simulink model "c00014M_harness"  (R2018a)
settings: Solver=FixedStepAuto  StartTime=0.0  StopTime=300  FixedStep=0.1  RelTol=1e-3
undefined symbols (not defined in the file): A1, hmax, PriorityTank, R1, R2, sigbuilder_block
(part 13 of 24)

== system c00014M_harness/M144/Tank1/Control ==
  note: 1: Maintenance
      | 2: Reference
      | 3: Manual
  ControlType : Inport
  Fill : Inport  Port=2
  Empty : Inport  Port=3
  EmergencyButton : Inport  Port=4
  LiquidLevel : Inport  Port=5
  Constant : Constant  Value=0
  ManualControlLiquidInOut : Subsystem
  Switch : Switch  Criteria=u2 > Threshold
  Switch1 : Switch  Criteria=u2 > Threshold
  LiquidIn : Outport
  LiquidOut : Outport  Port=2
  wires:
  LiquidLevel/1 -> ManualControlLiquidInOut/3(LiquidLevel)
  Empty/1 -> ManualControlLiquidInOut/2(Empty)
  Fill/1 -> ManualControlLiquidInOut/1(Fill)
  Switch/1 -> LiquidIn/1
  Switch1/1 -> LiquidOut/1
  Constant/1 -> Switch1/1, Switch/1
  EmergencyButton/1 -> Switch/2, Switch1/2
  ManualControlLiquidInOut/1(LiquidIn) -> Switch/3
  ManualControlLiquidInOut/2(LiquidOut) -> Switch1/3

== system c00014M_harness/M144/Tank1/MasterTankControl ==
  note: Priority tank must always have more liquid than others
  LiquidTank1 : Inport
  LiquidTank3 : Inport  Port=2
  Constant : Constant  Value=PriorityTank
  Constant1 : Constant  Value=false
  Logical Operator : Logic  Operator=NOT  AllPortsSameDT=off  OutDataTypeStr=boolean
  Multiport Switch : MultiPortSwitch
  Relational Operator1 : RelationalOperator  OutDataTypeStr=boolean  RndMeth=Simplest
  AllowTheTankFilling : Outport
  wires:
  LiquidTank3/1 -> Relational Operator1/2
  LiquidTank1/1 -> Relational Operator1/1
  Constant/1 -> Multiport Switch/1
  Relational Operator1/1 -> Multiport Switch/4
  Constant1/1 -> Multiport Switch/2, Multiport Switch/3
  Multiport Switch/1 -> Logical Operator/1
  Logical Operator/1 -> AllowTheTankFilling/1

== system c00014M_harness/M144/Tank1/TankModel ==
  LiquidIn : Inport
  LiquidOut : Inport  Port=2
  Add1 : Sum  Inputs=+-
  Constant1 : Constant  Value=0
  Constant2 : Constant  Value=0
  Constant3 : Constant
  Gain : Gain  Gain=1/R1
  Gain1 : Gain  Gain=1/A1
  Gain2 : Gain  Gain=1/R2
  Integrator : Integrator
  Saturation : Saturate  UpperLimit=hmax  LowerLimit=0
  Switch : Switch  Criteria=u2 ~= 0
  Switch1 : Switch  Criteria=u2 ~= 0
  LiquidLevel : Outport
  wires:
  Saturation/1 -> LiquidLevel/1, Gain2/1
  LiquidOut/1 -> Switch/2
  Add1/1 -> Gain1/1
  Gain2/1 -> Switch/1
  LiquidIn/1 -> Switch1/2
  Switch/1 -> Add1/2
  Switch1/1 -> Gain/1
  Constant2/1 -> Switch/3
  Constant3/1 -> Switch1/1
  Integrator/1 -> Saturation/1
  Gain1/1 -> Integrator/1
  Gain/1 -> Add1/1
  Constant1/1 -> Switch1/3

== system c00014M_harness/M144/Tank3/Control ==
  note: 1: Maintenance
      | 2: Reference
      | 3: Manual
  ControlType : Inport
  StartMaintenance : Inport  Port=2
  EmergencyButton : Inport  Port=3
  LiquidLevel : Inport  Port=4
  Constant : Constant  Value=0
  Maintenance : Subsystem
  Switch : Switch  Criteria=u2 > Threshold
  Switch1 : Switch  Criteria=u2 > Threshold
  LiquidIn : Outport
  LiquidOut : Outport  Port=2
  wires:
  ControlType/1 -> Maintenance/1(Type)
  LiquidLevel/1 -> Maintenance/3(LiquidLevel)
  StartMaintenance/1 -> Maintenance/2(StartMaintenance)
  Switch/1 -> LiquidIn/1
  Switch1/1 -> LiquidOut/1
  Constant/1 -> Switch1/1, Switch/1
  EmergencyButton/1 -> Switch/2, Switch1/2
  Maintenance/1(LiquidIn) -> Switch/3
  Maintenance/2(LiquidOut) -> Switch1/3

== system c00014M_harness/M144/Tank3/MasterTankControl ==
  note: Priority tank must always have more liquid than others
  LiquidTank1 : Inport
  LiquidTank3 : Inport  Port=2
  Constant : Constant  Value=PriorityTank
  Constant1 : Constant  Value=false
  Logical Operator : Logic  Operator=NOT  AllPortsSameDT=off  OutDataTypeStr=boolean
  Multiport Switch : MultiPortSwitch
  Relational Operator : RelationalOperator  OutDataTypeStr=boolean  RndMeth=Simplest
  AllowTheTankFilling : Outport
  wires:
  Constant/1 -> Multiport Switch/1
  Relational Operator/1 -> Multiport Switch/2
  Constant1/1 -> Multiport Switch/4, Multiport Switch/3
  Multiport Switch/1 -> Logical Operator/1
  Logical Operator/1 -> AllowTheTankFilling/1
  LiquidTank1/1 -> Relational Operator/2
  LiquidTank3/1 -> Relational Operator/1

== system c00014M_harness/M144/Tank3/TankModel ==
  LiquidIn : Inport
  LiquidOut : Inport  Port=2
  Add1 : Sum  Inputs=+-
  Constant1 : Constant  Value=0
  Constant2 : Constant  Value=0
  Constant3 : Constant
  Gain : Gain  Gain=1/R1
  Gain1 : Gain  Gain=1/A1
  Gain2 : Gain  Gain=1/R2
  Integrator : Integrator
  Saturation : Saturate  UpperLimit=hmax  LowerLimit=0
  Switch : Switch  Criteria=u2 ~= 0
  Switch1 : Switch  Criteria=u2 ~= 0
  LiquidLevel : Outport
  wires:
  Saturation/1 -> LiquidLevel/1, Gain2/1
  LiquidOut/1 -> Switch/2
  Add1/1 -> Gain1/1
  Gain2/1 -> Switch/1
  LiquidIn/1 -> Switch1/2
  Switch/1 -> Add1/2
  Switch1/1 -> Gain/1
  Constant2/1 -> Switch/3
  Constant3/1 -> Switch1/1
  Integrator/1 -> Saturation/1
  Gain1/1 -> Integrator/1
  Gain/1 -> Add1/1
  Constant1/1 -> Switch1/3

== system c00014M_harness/M145/Tank1/Control ==
  note: 1: Maintenance
      | 2: Reference
      | 3: Manual
  ControlType : Inport
  Fill : Inport  Port=2
  Empty : Inport  Port=3
  EmergencyButton : Inport  Port=4
  LiquidLevel : Inport  Port=5
  Constant : Constant  Value=0
  ManualControlLiquidInOut : Subsystem
  Switch : Switch  Criteria=u2 > Threshold
  Switch1 : Switch  Criteria=u2 > Threshold
  LiquidIn : Outport
  LiquidOut : Outport  Port=2
  wires:
  LiquidLevel/1 -> ManualControlLiquidInOut/3(LiquidLevel)
  Empty/1 -> ManualControlLiquidInOut/2(Empty)
  Fill/1 -> ManualControlLiquidInOut/1(Fill)
  Switch/1 -> LiquidIn/1
  Switch1/1 -> LiquidOut/1
  Constant/1 -> Switch1/1, Switch/1
  EmergencyButton/1 -> Switch/2, Switch1/2
  ManualControlLiquidInOut/1(LiquidIn) -> Switch/3
  ManualControlLiquidInOut/2(LiquidOut) -> Switch1/3

== system c00014M_harness/M145/Tank1/MasterTankControl ==
  note: Priority tank must always have more liquid than others
  LiquidTank1 : Inport
  LiquidTank3 : Inport  Port=2
  Constant : Constant  Value=PriorityTank
  Constant1 : Constant  Value=false
  Logical Operator : Logic  Operator=NOT  AllPortsSameDT=off  OutDataTypeStr=boolean
  Multiport Switch : MultiPortSwitch
  Relational Operator1 : RelationalOperator  OutDataTypeStr=boolean  RndMeth=Simplest
  AllowTheTankFilling : Outport
  wires:
  LiquidTank3/1 -> Relational Operator1/2
  LiquidTank1/1 -> Relational Operator1/1
  Constant/1 -> Multiport Switch/1
  Relational Operator1/1 -> Multiport Switch/4
  Constant1/1 -> Multiport Switch/2, Multiport Switch/3
  Multiport Switch/1 -> Logical Operator/1
  Logical Operator/1 -> AllowTheTankFilling/1

== system c00014M_harness/M145/Tank1/TankModel ==
  LiquidIn : Inport
  LiquidOut : Inport  Port=2
  Add1 : Sum  Inputs=+-
  Constant1 : Constant  Value=0
  Constant2 : Constant  Value=0
  Constant3 : Constant
  Gain : Gain  Gain=1/R1
  Gain1 : Gain  Gain=1/A1
  Gain2 : Gain  Gain=1/R2
  Integrator : Integrator
  Saturation : Saturate  UpperLimit=hmax  LowerLimit=0
  Switch : Switch  Criteria=u2 ~= 0
  Switch1 : Switch  Criteria=u2 ~= 0
  LiquidLevel : Outport
  wires:
  Saturation/1 -> LiquidLevel/1, Gain2/1
  LiquidOut/1 -> Switch/2
  Add1/1 -> Gain1/1
  Gain2/1 -> Switch/1
  LiquidIn/1 -> Switch1/2
  Switch/1 -> Add1/2
  Switch1/1 -> Gain/1
  Constant2/1 -> Switch/3
  Constant3/1 -> Switch1/1
  Integrator/1 -> Saturation/1
  Gain1/1 -> Integrator/1
  Gain/1 -> Add1/1
  Constant1/1 -> Switch1/3

== system c00014M_harness/M145/Tank3/Control ==
  note: 1: Maintenance
      | 2: Reference
      | 3: Manual
  ControlType : Inport
  StartMaintenance : Inport  Port=2
  EmergencyButton : Inport  Port=3
  LiquidLevel : Inport  Port=4
  Constant : Constant  Value=0
  Maintenance : Subsystem
  Switch : Switch  Criteria=u2 > Threshold
  Switch1 : Switch  Criteria=u2 > Threshold
  LiquidIn : Outport
  LiquidOut : Outport  Port=2
  wires:
  ControlType/1 -> Maintenance/1(Type)
  LiquidLevel/1 -> Maintenance/3(LiquidLevel)
  StartMaintenance/1 -> Maintenance/2(StartMaintenance)
  Switch/1 -> LiquidIn/1
  Switch1/1 -> LiquidOut/1
  Constant/1 -> Switch1/1, Switch/1
  EmergencyButton/1 -> Switch/2, Switch1/2
  Maintenance/1(LiquidIn) -> Switch/3
  Maintenance/2(LiquidOut) -> Switch1/3

== system c00014M_harness/M145/Tank3/MasterTankControl ==
  note: Priority tank must always have more liquid than others
  LiquidTank1 : Inport
  LiquidTank3 : Inport  Port=2
  Constant : Constant  Value=PriorityTank
  Constant1 : Constant  Value=false
  Logical Operator : Logic  Operator=NOT  AllPortsSameDT=off  OutDataTypeStr=boolean
  Multiport Switch : MultiPortSwitch
  Relational Operator : RelationalOperator  OutDataTypeStr=boolean  RndMeth=Simplest
  AllowTheTankFilling : Outport
  wires:
  Constant/1 -> Multiport Switch/1
  Relational Operator/1 -> Multiport Switch/2
  Constant1/1 -> Multiport Switch/4, Multiport Switch/3
  Multiport Switch/1 -> Logical Operator/1
  Logical Operator/1 -> AllowTheTankFilling/1
  LiquidTank1/1 -> Relational Operator/2
  LiquidTank3/1 -> Relational Operator/1

== system c00014M_harness/M145/Tank3/TankModel ==
  LiquidIn : Inport
  LiquidOut : Inport  Port=2
  Add1 : Sum  Inputs=+-
  Constant1 : Constant  Value=0
  Constant2 : Constant  Value=0
  Constant3 : Constant
  Gain : Gain  Gain=1/R1
  Gain1 : Gain  Gain=1/A1
  Gain2 : Gain  Gain=1/R2
  Integrator : Integrator
  Saturation : Saturate  UpperLimit=hmax  LowerLimit=0
  Switch : Switch  Criteria=u2 ~= 0
  Switch1 : Switch  Criteria=u2 ~= 0
  LiquidLevel : Outport
  wires:
  Saturation/1 -> LiquidLevel/1, Gain2/1
  LiquidOut/1 -> Switch/2
  Add1/1 -> Gain1/1
  Gain2/1 -> Switch/1
  LiquidIn/1 -> Switch1/2
  Switch/1 -> Add1/2
  Switch1/1 -> Gain/1
  Constant2/1 -> Switch/3
  Constant3/1 -> Switch1/1
  Integrator/1 -> Saturation/1
  Gain1/1 -> Integrator/1
  Gain/1 -> Add1/1
  Constant1/1 -> Switch1/3

== system c00014M_harness/M146/Tank1/Control ==
  note: 1: Maintenance
      | 2: Reference
      | 3: Manual
  ControlType : Inport
  Fill : Inport  Port=2
  Empty : Inport  Port=3
  EmergencyButton : Inport  Port=4
  LiquidLevel : Inport  Port=5
  Constant : Constant  Value=0
  ManualControlLiquidInOut : Subsystem
  Switch : Switch  Criteria=u2 > Threshold
  Switch1 : Switch  Criteria=u2 > Threshold
  LiquidIn : Outport
  LiquidOut : Outport  Port=2
  wires:
  LiquidLevel/1 -> ManualControlLiquidInOut/3(LiquidLevel)
  Empty/1 -> ManualControlLiquidInOut/2(Empty)
  Fill/1 -> ManualControlLiquidInOut/1(Fill)
  Switch/1 -> LiquidIn/1
  Switch1/1 -> LiquidOut/1
  Constant/1 -> Switch1/1, Switch/1
  EmergencyButton/1 -> Switch/2, Switch1/2
  ManualControlLiquidInOut/1(LiquidIn) -> Switch/3
  ManualControlLiquidInOut/2(LiquidOut) -> Switch1/3

== system c00014M_harness/M146/Tank1/MasterTankControl ==
  note: Priority tank must always have more liquid than others
  LiquidTank1 : Inport
  LiquidTank3 : Inport  Port=2
  Constant : Constant  Value=PriorityTank
  Constant1 : Constant  Value=false
  Logical Operator : Logic  Operator=NOT  AllPortsSameDT=off  OutDataTypeStr=boolean
  Multiport Switch : MultiPortSwitch
  Relational Operator1 : RelationalOperator  OutDataTypeStr=boolean  RndMeth=Simplest
  AllowTheTankFilling : Outport
  wires:
  LiquidTank3/1 -> Relational Operator1/2
  LiquidTank1/1 -> Relational Operator1/1
  Constant/1 -> Multiport Switch/1
  Relational Operator1/1 -> Multiport Switch/4
  Constant1/1 -> Multiport Switch/2, Multiport Switch/3
  Multiport Switch/1 -> Logical Operator/1
  Logical Operator/1 -> AllowTheTankFilling/1

== system c00014M_harness/M146/Tank1/TankModel ==
  LiquidIn : Inport
  LiquidOut : Inport  Port=2
  Add1 : Sum  Inputs=+-
  Constant1 : Constant  Value=0
  Constant2 : Constant  Value=0
  Constant3 : Constant
  Gain : Gain  Gain=1/R1
  Gain1 : Gain  Gain=1/A1
  Gain2 : Gain  Gain=1/R2
  Integrator : Integrator
  Saturation : Saturate  UpperLimit=hmax  LowerLimit=0
  Switch : Switch  Criteria=u2 ~= 0
  Switch1 : Switch  Criteria=u2 ~= 0
  LiquidLevel : Outport
  wires:
  Saturation/1 -> LiquidLevel/1, Gain2/1
  LiquidOut/1 -> Switch/2
  Add1/1 -> Gain1/1
  Gain2/1 -> Switch/1
  LiquidIn/1 -> Switch1/2
  Switch/1 -> Add1/2
  Switch1/1 -> Gain/1
  Constant2/1 -> Switch/3
  Constant3/1 -> Switch1/1
  Integrator/1 -> Saturation/1
  Gain1/1 -> Integrator/1
  Gain/1 -> Add1/1
  Constant1/1 -> Switch1/3

== system c00014M_harness/M146/Tank3/Control ==
  note: 1: Maintenance
      | 2: Reference
      | 3: Manual
  ControlType : Inport
  StartMaintenance : Inport  Port=2
  EmergencyButton : Inport  Port=3
  LiquidLevel : Inport  Port=4
  Constant : Constant  Value=0
  Maintenance : Subsystem
  Switch : Switch  Criteria=u2 > Threshold
  Switch1 : Switch  Criteria=u2 > Threshold
  LiquidIn : Outport
  LiquidOut : Outport  Port=2
  wires:
  ControlType/1 -> Maintenance/1(Type)
  LiquidLevel/1 -> Maintenance/3(LiquidLevel)
  StartMaintenance/1 -> Maintenance/2(StartMaintenance)
  Switch/1 -> LiquidIn/1
  Switch1/1 -> LiquidOut/1
  Constant/1 -> Switch1/1, Switch/1
  EmergencyButton/1 -> Switch/2, Switch1/2
  Maintenance/1(LiquidIn) -> Switch/3
  Maintenance/2(LiquidOut) -> Switch1/3

== system c00014M_harness/M146/Tank3/MasterTankControl ==
  note: Priority tank must always have more liquid than others
  LiquidTank1 : Inport
  LiquidTank3 : Inport  Port=2
  Constant : Constant  Value=PriorityTank
  Constant1 : Constant  Value=false
  Logical Operator : Logic  Operator=NOT  AllPortsSameDT=off  OutDataTypeStr=boolean
  Multiport Switch : MultiPortSwitch
  Relational Operator : RelationalOperator  OutDataTypeStr=boolean  RndMeth=Simplest
  AllowTheTankFilling : Outport
  wires:
  Constant/1 -> Multiport Switch/1
  Relational Operator/1 -> Multiport Switch/2
  Constant1/1 -> Multiport Switch/4, Multiport Switch/3
  Multiport Switch/1 -> Logical Operator/1
  Logical Operator/1 -> AllowTheTankFilling/1
  LiquidTank1/1 -> Relational Operator/2
  LiquidTank3/1 -> Relational Operator/1

== system c00014M_harness/M146/Tank3/TankModel ==
  LiquidIn : Inport
  LiquidOut : Inport  Port=2
  Add1 : Sum  Inputs=+-
  Constant1 : Constant  Value=0
  Constant2 : Constant  Value=0
  Constant3 : Constant
  Gain : Gain  Gain=1/R1
  Gain1 : Gain  Gain=1/A1
  Gain2 : Gain  Gain=1/R2
  Integrator : Integrator
  Saturation : Saturate  UpperLimit=hmax  LowerLimit=0
  Switch : Switch  Criteria=u2 ~= 0
  Switch1 : Switch  Criteria=u2 ~= 0
  LiquidLevel : Outport
  wires:
  Saturation/1 -> LiquidLevel/1, Gain2/1
  LiquidOut/1 -> Switch/2
  Add1/1 -> Gain1/1
  Gain2/1 -> Switch/1
  LiquidIn/1 -> Switch1/2
  Switch/1 -> Add1/2
  Switch1/1 -> Gain/1
  Constant2/1 -> Switch/3
  Constant3/1 -> Switch1/1
  Integrator/1 -> Saturation/1
  Gain1/1 -> Integrator/1
  Gain/1 -> Add1/1
  Constant1/1 -> Switch1/3

== system c00014M_harness/M147/Tank1/Control ==
  note: 1: Maintenance
      | 2: Reference
      | 3: Manual
  ControlType : Inport
  Fill : Inport  Port=2
  Empty : Inport  Port=3
  EmergencyButton : Inport  Port=4
  LiquidLevel : Inport  Port=5
  Constant : Constant  Value=0
  ManualControlLiquidInOut : Subsystem
  Switch : Switch  Criteria=u2 > Threshold
  Switch1 : Switch  Criteria=u2 > Threshold
  LiquidIn : Outport
  LiquidOut : Outport  Port=2
  wires:
  LiquidLevel/1 -> ManualControlLiquidInOut/3(LiquidLevel)
  Empty/1 -> ManualControlLiquidInOut/2(Empty)
  Fill/1 -> ManualControlLiquidInOut/1(Fill)
  Switch/1 -> LiquidIn/1
  Switch1/1 -> LiquidOut/1
  Constant/1 -> Switch1/1, Switch/1
  EmergencyButton/1 -> Switch/2, Switch1/2
  ManualControlLiquidInOut/1(LiquidIn) -> Switch/3
  ManualControlLiquidInOut/2(LiquidOut) -> Switch1/3

== system c00014M_harness/M147/Tank1/MasterTankControl ==
  note: Priority tank must always have more liquid than others
  LiquidTank1 : Inport
  LiquidTank3 : Inport  Port=2
  Constant : Constant  Value=PriorityTank
  Constant1 : Constant  Value=false
  Logical Operator : Logic  Operator=NOT  AllPortsSameDT=off  OutDataTypeStr=boolean
  Multiport Switch : MultiPortSwitch
  Relational Operator1 : RelationalOperator  OutDataTypeStr=boolean  RndMeth=Simplest
  AllowTheTankFilling : Outport
  wires:
  LiquidTank3/1 -> Relational Operator1/2
  LiquidTank1/1 -> Relational Operator1/1
  Constant/1 -> Multiport Switch/1
  Relational Operator1/1 -> Multiport Switch/4
  Constant1/1 -> Multiport Switch/2, Multiport Switch/3
  Multiport Switch/1 -> Logical Operator/1
  Logical Operator/1 -> AllowTheTankFilling/1

== system c00014M_harness/M147/Tank1/TankModel ==
  LiquidIn : Inport
  LiquidOut : Inport  Port=2
  Add1 : Sum  Inputs=+-
  Constant1 : Constant  Value=0
  Constant2 : Constant  Value=0
  Constant3 : Constant
  Gain : Gain  Gain=1/R1
  Gain1 : Gain  Gain=1/A1
  Gain2 : Gain  Gain=1/R2
  Integrator : Integrator
  Saturation : Saturate  UpperLimit=hmax  LowerLimit=0
  Switch : Switch  Criteria=u2 ~= 0
  Switch1 : Switch  Criteria=u2 ~= 0
  LiquidLevel : Outport
  wires:
  Saturation/1 -> LiquidLevel/1, Gain2/1
  LiquidOut/1 -> Switch/2
  Add1/1 -> Gain1/1
  Gain2/1 -> Switch/1
  LiquidIn/1 -> Switch1/2
  Switch/1 -> Add1/2
  Switch1/1 -> Gain/1
  Constant2/1 -> Switch/3
  Constant3/1 -> Switch1/1
  Integrator/1 -> Saturation/1
  Gain1/1 -> Integrator/1
  Gain/1 -> Add1/1
  Constant1/1 -> Switch1/3

== system c00014M_harness/M147/Tank3/Control ==
  note: 1: Maintenance
      | 2: Reference
      | 3: Manual
  ControlType : Inport
  StartMaintenance : Inport  Port=2
  EmergencyButton : Inport  Port=3
  LiquidLevel : Inport  Port=4
  Constant : Constant  Value=0
  Maintenance : Subsystem
  Switch : Switch  Criteria=u2 > Threshold
  Switch1 : Switch  Criteria=u2 > Threshold
  LiquidIn : Outport
  LiquidOut : Outport  Port=2
  wires:
  ControlType/1 -> Maintenance/1(Type)
  LiquidLevel/1 -> Maintenance/3(LiquidLevel)
  StartMaintenance/1 -> Maintenance/2(StartMaintenance)
  Switch/1 -> LiquidIn/1
  Switch1/1 -> LiquidOut/1
  Constant/1 -> Switch1/1, Switch/1
  EmergencyButton/1 -> Switch/2, Switch1/2
  Maintenance/1(LiquidIn) -> Switch/3
  Maintenance/2(LiquidOut) -> Switch1/3

== system c00014M_harness/M147/Tank3/MasterTankControl ==
  note: Priority tank must always have more liquid than others
  LiquidTank1 : Inport
  LiquidTank3 : Inport  Port=2
  Constant : Constant  Value=PriorityTank
  Constant1 : Constant  Value=false
  Logical Operator : Logic  Operator=NOT  AllPortsSameDT=off  OutDataTypeStr=boolean
  Multiport Switch : MultiPortSwitch
  Relational Operator : RelationalOperator  OutDataTypeStr=boolean  RndMeth=Simplest
  AllowTheTankFilling : Outport
  wires:
  Constant/1 -> Multiport Switch/1
  Relational Operator/1 -> Multiport Switch/2
  Constant1/1 -> Multiport Switch/4, Multiport Switch/3
  Multiport Switch/1 -> Logical Operator/1
  Logical Operator/1 -> AllowTheTankFilling/1
  LiquidTank1/1 -> Relational Operator/2
  LiquidTank3/1 -> Relational Operator/1

== system c00014M_harness/M147/Tank3/TankModel ==
  LiquidIn : Inport
  LiquidOut : Inport  Port=2
  Add1 : Sum  Inputs=+-
  Constant1 : Constant  Value=0
  Constant2 : Constant  Value=0
  Constant3 : Constant
  Gain : Gain  Gain=1/R1
  Gain1 : Gain  Gain=1/A1
  Gain2 : Gain  Gain=1/R2
  Integrator : Integrator
  Saturation : Saturate  UpperLimit=hmax  LowerLimit=0
  Switch : Switch  Criteria=u2 ~= 0
  Switch1 : Switch  Criteria=u2 ~= 0
  LiquidLevel : Outport
  wires:
  Saturation/1 -> LiquidLevel/1, Gain2/1
  LiquidOut/1 -> Switch/2
  Add1/1 -> Gain1/1
  Gain2/1 -> Switch/1
  LiquidIn/1 -> Switch1/2
  Switch/1 -> Add1/2
  Switch1/1 -> Gain/1
  Constant2/1 -> Switch/3
  Constant3/1 -> Switch1/1
  Integrator/1 -> Saturation/1
  Gain1/1 -> Integrator/1
  Gain/1 -> Add1/1
  Constant1/1 -> Switch1/3

== system c00014M_harness/M148/Tank1/Control ==
  note: 1: Maintenance
      | 2: Reference
      | 3: Manual
  ControlType : Inport
  Fill : Inport  Port=2
  Empty : Inport  Port=3
  EmergencyButton : Inport  Port=4
  LiquidLevel : Inport  Port=5
  Constant : Constant  Value=0
  ManualControlLiquidInOut : Subsystem
  Switch : Switch  Criteria=u2 > Threshold
  Switch1 : Switch  Criteria=u2 > Threshold
  LiquidIn : Outport
  LiquidOut : Outport  Port=2
  wires:
  LiquidLevel/1 -> ManualControlLiquidInOut/3(LiquidLevel)
  Empty/1 -> ManualControlLiquidInOut/2(Empty)
  Fill/1 -> ManualControlLiquidInOut/1(Fill)
  Switch/1 -> LiquidIn/1
  Switch1/1 -> LiquidOut/1
  Constant/1 -> Switch1/1, Switch/1
  EmergencyButton/1 -> Switch/2, Switch1/2
  ManualControlLiquidInOut/1(LiquidIn) -> Switch/3
  ManualControlLiquidInOut/2(LiquidOut) -> Switch1/3

== system c00014M_harness/M148/Tank1/MasterTankControl ==
  note: Priority tank must always have more liquid than others
  LiquidTank1 : Inport
  LiquidTank3 : Inport  Port=2
  Constant : Constant  Value=PriorityTank
  Constant1 : Constant  Value=false
  Logical Operator : Logic  Operator=NOT  AllPortsSameDT=off  OutDataTypeStr=boolean
  Multiport Switch : MultiPortSwitch
  Relational Operator1 : RelationalOperator  OutDataTypeStr=boolean  RndMeth=Simplest
  AllowTheTankFilling : Outport
  wires:
  LiquidTank3/1 -> Relational Operator1/2
  LiquidTank1/1 -> Relational Operator1/1
  Constant/1 -> Multiport Switch/1
  Relational Operator1/1 -> Multiport Switch/4
  Constant1/1 -> Multiport Switch/2, Multiport Switch/3
  Multiport Switch/1 -> Logical Operator/1
  Logical Operator/1 -> AllowTheTankFilling/1

== system c00014M_harness/M148/Tank1/TankModel ==
  LiquidIn : Inport
  LiquidOut : Inport  Port=2
  Add1 : Sum  Inputs=+-
  Constant1 : Constant  Value=0
  Constant2 : Constant  Value=0
  Constant3 : Constant
  Gain : Gain  Gain=1/R1
  Gain1 : Gain  Gain=1/A1
  Gain2 : Gain  Gain=1/R2
  Integrator : Integrator
  Saturation : Saturate  UpperLimit=hmax  LowerLimit=0
  Switch : Switch  Criteria=u2 ~= 0
  Switch1 : Switch  Criteria=u2 ~= 0
  LiquidLevel : Outport
  wires:
  Saturation/1 -> LiquidLevel/1, Gain2/1
  LiquidOut/1 -> Switch/2
  Add1/1 -> Gain1/1
  Gain2/1 -> Switch/1
  LiquidIn/1 -> Switch1/2
  Switch/1 -> Add1/2
  Switch1/1 -> Gain/1
  Constant2/1 -> Switch/3
  Constant3/1 -> Switch1/1
  Integrator/1 -> Saturation/1
  Gain1/1 -> Integrator/1
  Gain/1 -> Add1/1
  Constant1/1 -> Switch1/3

== system c00014M_harness/M148/Tank3/Control ==
  note: 1: Maintenance
      | 2: Reference
      | 3: Manual
  ControlType : Inport
  StartMaintenance : Inport  Port=2
  EmergencyButton : Inport  Port=3
  LiquidLevel : Inport  Port=4
  Constant : Constant  Value=0
  Maintenance : Subsystem
  Switch : Switch  Criteria=u2 > Threshold
  Switch1 : Switch  Criteria=u2 > Threshold
  LiquidIn : Outport
  LiquidOut : Outport  Port=2
  wires:
  ControlType/1 -> Maintenance/1(Type)
  LiquidLevel/1 -> Maintenance/3(LiquidLevel)
  StartMaintenance/1 -> Maintenance/2(StartMaintenance)
  Switch/1 -> LiquidIn/1
  Switch1/1 -> LiquidOut/1
  Constant/1 -> Switch1/1, Switch/1
  EmergencyButton/1 -> Switch/2, Switch1/2
  Maintenance/1(LiquidIn) -> Switch/3
  Maintenance/2(LiquidOut) -> Switch1/3

== system c00014M_harness/M148/Tank3/MasterTankControl ==
  note: Priority tank must always have more liquid than others
  LiquidTank1 : Inport
  LiquidTank3 : Inport  Port=2
  Constant : Constant  Value=PriorityTank
  Constant1 : Constant  Value=false
  Logical Operator : Logic  Operator=NOT  AllPortsSameDT=off  OutDataTypeStr=boolean
  Multiport Switch : MultiPortSwitch
  Relational Operator : RelationalOperator  OutDataTypeStr=boolean  RndMeth=Simplest
  AllowTheTankFilling : Outport
  wires:
  Constant/1 -> Multiport Switch/1
  Relational Operator/1 -> Multiport Switch/2
  Constant1/1 -> Multiport Switch/4, Multiport Switch/3
  Multiport Switch/1 -> Logical Operator/1
  Logical Operator/1 -> AllowTheTankFilling/1
  LiquidTank1/1 -> Relational Operator/2
  LiquidTank3/1 -> Relational Operator/1

== system c00014M_harness/M148/Tank3/TankModel ==
  LiquidIn : Inport
  LiquidOut : Inport  Port=2
  Add1 : Sum  Inputs=+-
  Constant1 : Constant  Value=0
  Constant2 : Constant  Value=0
  Constant3 : Constant
  Gain : Gain  Gain=1/R1
  Gain1 : Gain  Gain=1/A1
  Gain2 : Gain  Gain=1/R2
  Integrator : Integrator
  Saturation : Saturate  UpperLimit=hmax  LowerLimit=0
  Switch : Switch  Criteria=u2 ~= 0
  Switch1 : Switch  Criteria=u2 ~= 0
  LiquidLevel : Outport
  wires:
  Saturation/1 -> LiquidLevel/1, Gain2/1
  LiquidOut/1 -> Switch/2
  Add1/1 -> Gain1/1
  Gain2/1 -> Switch/1
  LiquidIn/1 -> Switch1/2
  Switch/1 -> Add1/2
  Switch1/1 -> Gain/1
  Constant2/1 -> Switch/3
  Constant3/1 -> Switch1/1
  Integrator/1 -> Saturation/1
  Gain1/1 -> Integrator/1
  Gain/1 -> Add1/1
  Constant1/1 -> Switch1/3

== system c00014M_harness/M165/Tank1/Control ==
  note: 1: Maintenance
      | 2: Reference
      | 3: Manual
  ControlType : Inport
  Fill : Inport  Port=2
  Empty : Inport  Port=3
  EmergencyButton : Inport  Port=4
  LiquidLevel : Inport  Port=5
  Constant : Constant  Value=0
  ManualControlLiquidInOut : Subsystem
  Switch : Switch  Criteria=u2 > Threshold
  Switch1 : Switch  Criteria=u2 > Threshold
  LiquidIn : Outport
  LiquidOut : Outport  Port=2
  wires:
  LiquidLevel/1 -> ManualControlLiquidInOut/3(LiquidLevel)
  Empty/1 -> ManualControlLiquidInOut/2(Empty)
  Fill/1 -> ManualControlLiquidInOut/1(Fill)
  Switch/1 -> LiquidIn/1
  Switch1/1 -> LiquidOut/1
  Constant/1 -> Switch1/1, Switch/1
  EmergencyButton/1 -> Switch/2, Switch1/2
  ManualControlLiquidInOut/1(LiquidIn) -> Switch/3
  ManualControlLiquidInOut/2(LiquidOut) -> Switch1/3

== system c00014M_harness/M165/Tank1/MasterTankControl ==
  note: Priority tank must always have more liquid than others
  LiquidTank1 : Inport
  LiquidTank3 : Inport  Port=2
  Constant : Constant  Value=PriorityTank
  Constant1 : Constant  Value=false
  Logical Operator : Logic  Operator=NOT  AllPortsSameDT=off  OutDataTypeStr=boolean
  Multiport Switch : MultiPortSwitch
  Relational Operator1 : RelationalOperator  OutDataTypeStr=boolean  RndMeth=Simplest
  AllowTheTankFilling : Outport
  wires:
  LiquidTank3/1 -> Relational Operator1/2
  LiquidTank1/1 -> Relational Operator1/1
  Constant/1 -> Multiport Switch/1
  Relational Operator1/1 -> Multiport Switch/4
  Constant1/1 -> Multiport Switch/2, Multiport Switch/3
  Multiport Switch/1 -> Logical Operator/1
  Logical Operator/1 -> AllowTheTankFilling/1

== system c00014M_harness/M165/Tank1/TankModel ==
  LiquidIn : Inport
  LiquidOut : Inport  Port=2
  Add1 : Sum  Inputs=+-
  Constant1 : Constant  Value=0
  Constant2 : Constant  Value=0
  Constant3 : Constant
  Gain : Gain  Gain=1/R1
  Gain1 : Gain  Gain=1/A1
  Gain2 : Gain  Gain=1/R2
  Integrator : Integrator
  Saturation : Saturate  UpperLimit=hmax  LowerLimit=0
  Switch : Switch  Criteria=u2 ~= 0
  Switch1 : Switch  Criteria=u2 ~= 0
  LiquidLevel : Outport
  wires:
  Saturation/1 -> LiquidLevel/1, Gain2/1
  LiquidOut/1 -> Switch/2
  Add1/1 -> Gain1/1
  Gain2/1 -> Switch/1
  LiquidIn/1 -> Switch1/2
  Switch/1 -> Add1/2
  Switch1/1 -> Gain/1
  Constant2/1 -> Switch/3
  Constant3/1 -> Switch1/1
  Integrator/1 -> Saturation/1
  Gain1/1 -> Integrator/1
  Gain/1 -> Add1/1
  Constant1/1 -> Switch1/3

== system c00014M_harness/M165/Tank3/Control ==
  note: 1: Maintenance
      | 2: Reference
      | 3: Manual
  ControlType : Inport
  StartMaintenance : Inport  Port=2
  EmergencyButton : Inport  Port=3
  LiquidLevel : Inport  Port=4
  Constant : Constant
  Maintenance : Subsystem
  Switch : Switch  Criteria=u2 > Threshold
  Switch1 : Switch  Criteria=u2 > Threshold
  LiquidIn : Outport
  LiquidOut : Outport  Port=2
  wires:
  ControlType/1 -> Maintenance/1(Type)
  LiquidLevel/1 -> Maintenance/3(LiquidLevel)
  StartMaintenance/1 -> Maintenance/2(StartMaintenance)
  Switch/1 -> LiquidIn/1
  Switch1/1 -> LiquidOut/1
  Constant/1 -> Switch1/1, Switch/1
  EmergencyButton/1 -> Switch/2, Switch1/2
  Maintenance/1(LiquidIn) -> Switch/3
  Maintenance/2(LiquidOut) -> Switch1/3

== system c00014M_harness/M165/Tank3/MasterTankControl ==
  note: Priority tank must always have more liquid than others
  LiquidTank1 : Inport
  LiquidTank3 : Inport  Port=2
  Constant : Constant  Value=PriorityTank
  Constant1 : Constant  Value=false
  Logical Operator : Logic  Operator=NOT  AllPortsSameDT=off  OutDataTypeStr=boolean
  Multiport Switch : MultiPortSwitch
  Relational Operator : RelationalOperator  OutDataTypeStr=boolean  RndMeth=Simplest
  AllowTheTankFilling : Outport
  wires:
  Constant/1 -> Multiport Switch/1
  Relational Operator/1 -> Multiport Switch/2
  Constant1/1 -> Multiport Switch/4, Multiport Switch/3
  Multiport Switch/1 -> Logical Operator/1
  Logical Operator/1 -> AllowTheTankFilling/1
  LiquidTank1/1 -> Relational Operator/2
  LiquidTank3/1 -> Relational Operator/1

== system c00014M_harness/M165/Tank3/TankModel ==
  LiquidIn : Inport
  LiquidOut : Inport  Port=2
  Add1 : Sum  Inputs=+-
  Constant1 : Constant  Value=0
  Constant2 : Constant  Value=0
  Constant3 : Constant
  Gain : Gain  Gain=1/R1
  Gain1 : Gain  Gain=1/A1
  Gain2 : Gain  Gain=1/R2
  Integrator : Integrator
  Saturation : Saturate  UpperLimit=hmax  LowerLimit=0
  Switch : Switch  Criteria=u2 ~= 0
  Switch1 : Switch  Criteria=u2 ~= 0
  LiquidLevel : Outport
  wires:
  Saturation/1 -> LiquidLevel/1, Gain2/1
  LiquidOut/1 -> Switch/2
  Add1/1 -> Gain1/1
  Gain2/1 -> Switch/1
  LiquidIn/1 -> Switch1/2
  Switch/1 -> Add1/2
  Switch1/1 -> Gain/1
  Constant2/1 -> Switch/3
  Constant3/1 -> Switch1/1
  Integrator/1 -> Saturation/1
  Gain1/1 -> Integrator/1
  Gain/1 -> Add1/1
  Constant1/1 -> Switch1/3

== system c00014M_harness/M169/Tank1/Control ==
  note: 1: Maintenance
      | 2: Reference
      | 3: Manual
  ControlType : Inport
  Fill : Inport  Port=2
  Empty : Inport  Port=3
  EmergencyButton : Inport  Port=4
  LiquidLevel : Inport  Port=5
  Constant : Constant  Value=0
  ManualControlLiquidInOut : Subsystem
  Switch : Switch  Criteria=u2 > Threshold
  Switch1 : Switch  Criteria=u2 > Threshold
  LiquidIn : Outport
  LiquidOut : Outport  Port=2
  wires:
  LiquidLevel/1 -> ManualControlLiquidInOut/3(LiquidLevel)
  Empty/1 -> ManualControlLiquidInOut/2(Empty)
  Fill/1 -> ManualControlLiquidInOut/1(Fill)
  Switch/1 -> LiquidIn/1
  Switch1/1 -> LiquidOut/1
  Constant/1 -> Switch1/1, Switch/1
  EmergencyButton/1 -> Switch/2, Switch1/2
  ManualControlLiquidInOut/1(LiquidIn) -> Switch/3
  ManualControlLiquidInOut/2(LiquidOut) -> Switch1/3

== system c00014M_harness/M169/Tank1/MasterTankControl ==
  note: Priority tank must always have more liquid than others
  LiquidTank1 : Inport
  LiquidTank3 : Inport  Port=2
  Constant : Constant  Value=PriorityTank
  Constant1 : Constant  Value=false
  Logical Operator : Logic  Operator=NOT  AllPortsSameDT=off  OutDataTypeStr=boolean
  Multiport Switch : MultiPortSwitch
  Relational Operator1 : RelationalOperator  OutDataTypeStr=boolean  RndMeth=Simplest
  AllowTheTankFilling : Outport
  wires:
  LiquidTank3/1 -> Relational Operator1/2
  LiquidTank1/1 -> Relational Operator1/1
  Constant/1 -> Multiport Switch/1
  Relational Operator1/1 -> Multiport Switch/4
  Constant1/1 -> Multiport Switch/2, Multiport Switch/3
  Multiport Switch/1 -> Logical Operator/1
  Logical Operator/1 -> AllowTheTankFilling/1

== system c00014M_harness/M169/Tank1/TankModel ==
  LiquidIn : Inport
  LiquidOut : Inport  Port=2
  Add1 : Sum  Inputs=+-
  Constant1 : Constant  Value=0
  Constant2 : Constant  Value=0
  Constant3 : Constant
  Gain : Gain  Gain=1/R1
  Gain1 : Gain  Gain=1/A1
  Gain2 : Gain  Gain=1/R2
  Integrator : Integrator
  Saturation : Saturate  UpperLimit=hmax  LowerLimit=0
  Switch : Switch  Criteria=u2 ~= 0
  Switch1 : Switch  Criteria=u2 ~= 0
  LiquidLevel : Outport
  wires:
  Saturation/1 -> LiquidLevel/1, Gain2/1
  LiquidOut/1 -> Switch/2
  Add1/1 -> Gain1/1
  Gain2/1 -> Switch/1
  LiquidIn/1 -> Switch1/2
  Switch/1 -> Add1/2
  Switch1/1 -> Gain/1
  Constant2/1 -> Switch/3
  Constant3/1 -> Switch1/1
  Integrator/1 -> Saturation/1
  Gain1/1 -> Integrator/1
  Gain/1 -> Add1/1
  Constant1/1 -> Switch1/3

== system c00014M_harness/M169/Tank3/Control ==
  note: 1: Maintenance
      | 2: Reference
      | 3: Manual
  ControlType : Inport
  StartMaintenance : Inport  Port=2
  EmergencyButton : Inport  Port=3
  LiquidLevel : Inport  Port=4
  Constant : Constant  Value=0
  Maintenance : Subsystem
  Switch : Switch  Criteria=u2 > Threshold
  Switch1 : Switch  Criteria=u2 > Threshold
  LiquidIn : Outport
  LiquidOut : Outport  Port=2
  wires:
  ControlType/1 -> Maintenance/1(Type)
  LiquidLevel/1 -> Maintenance/3(LiquidLevel)
  StartMaintenance/1 -> Maintenance/2(StartMaintenance)
  Switch/1 -> LiquidIn/1
  Switch1/1 -> LiquidOut/1
  Constant/1 -> Switch1/1, Switch/1
  EmergencyButton/1 -> Switch/2, Switch1/2
  Maintenance/1(LiquidIn) -> Switch/3
  Maintenance/2(LiquidOut) -> Switch1/3

== system c00014M_harness/M169/Tank3/MasterTankControl ==
  note: Priority tank must always have more liquid than others
  LiquidTank1 : Inport
  LiquidTank3 : Inport  Port=2
  Constant : Constant  Value=PriorityTank
  Constant1 : Constant  Value=false
  Logical Operator : Logic  Operator=NOT  AllPortsSameDT=off  OutDataTypeStr=boolean
  Multiport Switch : MultiPortSwitch
  Relational Operator : RelationalOperator  OutDataTypeStr=boolean  RndMeth=Simplest
  AllowTheTankFilling : Outport
  wires:
  Constant/1 -> Multiport Switch/1
  Relational Operator/1 -> Multiport Switch/2
  Constant1/1 -> Multiport Switch/4, Multiport Switch/3
  Multiport Switch/1 -> Logical Operator/1
  Logical Operator/1 -> AllowTheTankFilling/1
  LiquidTank1/1 -> Relational Operator/2
  LiquidTank3/1 -> Relational Operator/1

== system c00014M_harness/M169/Tank3/TankModel ==
  LiquidIn : Inport
  LiquidOut : Inport  Port=2
  Add1 : Sum  Inputs=+-
  Constant1 : Constant  Value=0
  Constant2 : Constant  Value=0
  Constant3 : Constant
  Gain : Gain  Gain=1/R1
  Gain1 : Gain  Gain=1/A1
  Gain2 : Gain  Gain=1/R2
  Integrator : Integrator
  Saturation : Saturate  UpperLimit=hmax  LowerLimit=0
  Switch : Switch  Criteria=u2 ~= 0
  Switch1 : Switch  Criteria=u2 ~= 0
  LiquidLevel : Outport
  wires:
  Saturation/1 -> LiquidLevel/1, Gain2/1
  LiquidOut/1 -> Switch/2
  Add1/1 -> Gain1/1
  Gain2/1 -> Switch/1
  LiquidIn/1 -> Switch1/2
  Switch/1 -> Add1/2
  Switch1/1 -> Gain/1
  Constant2/1 -> Switch/3
  Constant3/1 -> Switch1/1
  Integrator/1 -> Saturation/1
  Gain1/1 -> Integrator/1
  Gain/1 -> Add1/1
  Constant1/1 -> Switch1/3

== system c00014M_harness/M170/Tank1/Control ==
  note: 1: Maintenance
      | 2: Reference
      | 3: Manual
  ControlType : Inport
  Fill : Inport  Port=2
  Empty : Inport  Port=3
  EmergencyButton : Inport  Port=4
  LiquidLevel : Inport  Port=5
  Constant : Constant  Value=0
  ManualControlLiquidInOut : Subsystem
  Switch : Switch  Criteria=u2 > Threshold
  Switch1 : Switch  Criteria=u2 > Threshold
  LiquidIn : Outport
  LiquidOut : Outport  Port=2
  wires:
  LiquidLevel/1 -> ManualControlLiquidInOut/3(LiquidLevel)
  Empty/1 -> ManualControlLiquidInOut/2(Empty)
  Fill/1 -> ManualControlLiquidInOut/1(Fill)
  Switch/1 -> LiquidIn/1
  Switch1/1 -> LiquidOut/1
  Constant/1 -> Switch1/1, Switch/1
  EmergencyButton/1 -> Switch/2, Switch1/2
  ManualControlLiquidInOut/1(LiquidIn) -> Switch/3
  ManualControlLiquidInOut/2(LiquidOut) -> Switch1/3

== system c00014M_harness/M170/Tank1/MasterTankControl ==
  note: Priority tank must always have more liquid than others
  LiquidTank1 : Inport
  LiquidTank3 : Inport  Port=2
  Constant : Constant  Value=PriorityTank
  Constant1 : Constant  Value=false
  Logical Operator : Logic  Operator=NOT  AllPortsSameDT=off  OutDataTypeStr=boolean
  Multiport Switch : MultiPortSwitch
  Relational Operator1 : RelationalOperator  OutDataTypeStr=boolean  RndMeth=Simplest
  AllowTheTankFilling : Outport
  wires:
  LiquidTank3/1 -> Relational Operator1/2
  LiquidTank1/1 -> Relational Operator1/1
  Constant/1 -> Multiport Switch/1
  Relational Operator1/1 -> Multiport Switch/4
  Constant1/1 -> Multiport Switch/2, Multiport Switch/3
  Multiport Switch/1 -> Logical Operator/1
  Logical Operator/1 -> AllowTheTankFilling/1

== system c00014M_harness/M170/Tank1/TankModel ==
  LiquidIn : Inport
  LiquidOut : Inport  Port=2
  Add1 : Sum  Inputs=+-
  Constant1 : Constant  Value=0
  Constant2 : Constant  Value=0
  Constant3 : Constant
  Gain : Gain  Gain=1/R1
  Gain1 : Gain  Gain=1/A1
  Gain2 : Gain  Gain=1/R2
  Integrator : Integrator
  Saturation : Saturate  UpperLimit=hmax  LowerLimit=0
  Switch : Switch  Criteria=u2 ~= 0
  Switch1 : Switch  Criteria=u2 ~= 0
  LiquidLevel : Outport
  wires:
  Saturation/1 -> LiquidLevel/1, Gain2/1
  LiquidOut/1 -> Switch/2
  Add1/1 -> Gain1/1
  Gain2/1 -> Switch/1
  LiquidIn/1 -> Switch1/2
  Switch/1 -> Add1/2
  Switch1/1 -> Gain/1
  Constant2/1 -> Switch/3
  Constant3/1 -> Switch1/1
  Integrator/1 -> Saturation/1
  Gain1/1 -> Integrator/1
  Gain/1 -> Add1/1
  Constant1/1 -> Switch1/3

== system c00014M_harness/M170/Tank3/Control ==
  note: 1: Maintenance
      | 2: Reference
      | 3: Manual
  ControlType : Inport
  StartMaintenance : Inport  Port=2
  EmergencyButton : Inport  Port=3
  LiquidLevel : Inport  Port=4
  Constant : Constant  Value=0
  Maintenance : Subsystem
  Switch : Switch  Criteria=u2 > Threshold
  Switch1 : Switch  Criteria=u2 > Threshold
  LiquidIn : Outport
  LiquidOut : Outport  Port=2
  wires:
  ControlType/1 -> Maintenance/1(Type)
  LiquidLevel/1 -> Maintenance/3(LiquidLevel)
  StartMaintenance/1 -> Maintenance/2(StartMaintenance)
  Switch/1 -> LiquidIn/1
  Switch1/1 -> LiquidOut/1
  Constant/1 -> Switch1/1, Switch/1
  EmergencyButton/1 -> Switch/2, Switch1/2
  Maintenance/1(LiquidIn) -> Switch/3
  Maintenance/2(LiquidOut) -> Switch1/3

== system c00014M_harness/M170/Tank3/MasterTankControl ==
  note: Priority tank must always have more liquid than others
  LiquidTank1 : Inport
  LiquidTank3 : Inport  Port=2
  Constant : Constant  Value=PriorityTank
  Constant1 : Constant  Value=false
  Logical Operator : Logic  Operator=NOT  AllPortsSameDT=off  OutDataTypeStr=boolean
  Multiport Switch : MultiPortSwitch
  Relational Operator : RelationalOperator  OutDataTypeStr=boolean  RndMeth=Simplest
  AllowTheTankFilling : Outport
  wires:
  Constant/1 -> Multiport Switch/1
  Relational Operator/1 -> Multiport Switch/2
  Constant1/1 -> Multiport Switch/4, Multiport Switch/3
  Multiport Switch/1 -> Logical Operator/1
  Logical Operator/1 -> AllowTheTankFilling/1
  LiquidTank1/1 -> Relational Operator/2
  LiquidTank3/1 -> Relational Operator/1

== system c00014M_harness/M170/Tank3/TankModel ==
  LiquidIn : Inport
  LiquidOut : Inport  Port=2
  Add1 : Sum  Inputs=+-
  Constant1 : Constant  Value=0
  Constant2 : Constant  Value=0
  Constant3 : Constant
  Gain : Gain  Gain=1/R1
  Gain1 : Gain  Gain=1/A1
  Gain2 : Gain  Gain=1/R2
  Integrator : Integrator
  Saturation : Saturate  UpperLimit=hmax  LowerLimit=0
  Switch : Switch  Criteria=u2 ~= 0
  Switch1 : Switch  Criteria=u2 ~= 0
  LiquidLevel : Outport
  wires:
  Saturation/1 -> LiquidLevel/1, Gain2/1
  LiquidOut/1 -> Switch/2
  Add1/1 -> Gain1/1
  Gain2/1 -> Switch/1
  LiquidIn/1 -> Switch1/2
  Switch/1 -> Add1/2
  Switch1/1 -> Gain/1
  Constant2/1 -> Switch/3
  Constant3/1 -> Switch1/1
  Integrator/1 -> Saturation/1
  Gain1/1 -> Integrator/1
  Gain/1 -> Add1/1
  Constant1/1 -> Switch1/3

== system c00014M_harness/M171/Tank1/Control ==
  note: 1: Maintenance
      | 2: Reference
      | 3: Manual
  ControlType : Inport
  Fill : Inport  Port=2
  Empty : Inport  Port=3
  EmergencyButton : Inport  Port=4
  LiquidLevel : Inport  Port=5
  Constant : Constant  Value=0
  ManualControlLiquidInOut : Subsystem
  Switch : Switch  Criteria=u2 > Threshold
  Switch1 : Switch  Criteria=u2 > Threshold
  LiquidIn : Outport
  LiquidOut : Outport  Port=2
  wires:
  LiquidLevel/1 -> ManualControlLiquidInOut/3(LiquidLevel)
  Empty/1 -> ManualControlLiquidInOut/2(Empty)
  Fill/1 -> ManualControlLiquidInOut/1(Fill)
  Switch/1 -> LiquidIn/1
  Switch1/1 -> LiquidOut/1
  Constant/1 -> Switch1/1, Switch/1
  EmergencyButton/1 -> Switch/2, Switch1/2
  ManualControlLiquidInOut/1(LiquidIn) -> Switch/3
  ManualControlLiquidInOut/2(LiquidOut) -> Switch1/3

== system c00014M_harness/M171/Tank1/MasterTankControl ==
  note: Priority tank must always have more liquid than others
  LiquidTank1 : Inport
  LiquidTank3 : Inport  Port=2
  Constant : Constant  Value=PriorityTank
  Constant1 : Constant  Value=false
  Logical Operator : Logic  Operator=NOT  AllPortsSameDT=off  OutDataTypeStr=boolean
  Multiport Switch : MultiPortSwitch
  Relational Operator1 : RelationalOperator  OutDataTypeStr=boolean  RndMeth=Simplest
  AllowTheTankFilling : Outport
  wires:
  LiquidTank3/1 -> Relational Operator1/2
  LiquidTank1/1 -> Relational Operator1/1
  Constant/1 -> Multiport Switch/1
  Relational Operator1/1 -> Multiport Switch/4
  Constant1/1 -> Multiport Switch/2, Multiport Switch/3
  Multiport Switch/1 -> Logical Operator/1
  Logical Operator/1 -> AllowTheTankFilling/1

== system c00014M_harness/M171/Tank1/TankModel ==
  LiquidIn : Inport
  LiquidOut : Inport  Port=2
  Add1 : Sum  Inputs=+-
  Constant1 : Constant  Value=0
  Constant2 : Constant  Value=0
  Constant3 : Constant
  Gain : Gain  Gain=1/R1
  Gain1 : Gain  Gain=1/A1
  Gain2 : Gain  Gain=1/R2
  Integrator : Integrator
  Saturation : Saturate  UpperLimit=hmax  LowerLimit=0
  Switch : Switch  Criteria=u2 ~= 0
  Switch1 : Switch  Criteria=u2 ~= 0
  LiquidLevel : Outport
  wires:
  Saturation/1 -> LiquidLevel/1, Gain2/1
  LiquidOut/1 -> Switch/2
  Add1/1 -> Gain1/1
  Gain2/1 -> Switch/1
  LiquidIn/1 -> Switch1/2
  Switch/1 -> Add1/2
  Switch1/1 -> Gain/1
  Constant2/1 -> Switch/3
  Constant3/1 -> Switch1/1
  Integrator/1 -> Saturation/1
  Gain1/1 -> Integrator/1
  Gain/1 -> Add1/1
  Constant1/1 -> Switch1/3

== system c00014M_harness/M171/Tank3/Control ==
  note: 1: Maintenance
      | 2: Reference
      | 3: Manual
  ControlType : Inport
  StartMaintenance : Inport  Port=2
  EmergencyButton : Inport  Port=3
  LiquidLevel : Inport  Port=4
  Constant : Constant  Value=0
  Maintenance : Subsystem
  Switch : Switch  Criteria=u2 > Threshold
  Switch1 : Switch  Criteria=u2 > Threshold
  LiquidIn : Outport
  LiquidOut : Outport  Port=2
  wires:
  ControlType/1 -> Maintenance/1(Type)
  LiquidLevel/1 -> Maintenance/3(LiquidLevel)
  StartMaintenance/1 -> Maintenance/2(StartMaintenance)
  Switch/1 -> LiquidIn/1
  Switch1/1 -> LiquidOut/1
  Constant/1 -> Switch1/1, Switch/1
  EmergencyButton/1 -> Switch/2, Switch1/2
  Maintenance/1(LiquidIn) -> Switch/3
  Maintenance/2(LiquidOut) -> Switch1/3

== system c00014M_harness/M171/Tank3/MasterTankControl ==
  note: Priority tank must always have more liquid than others
  LiquidTank1 : Inport
  LiquidTank3 : Inport  Port=2
  Constant : Constant  Value=PriorityTank
  Constant1 : Constant  Value=false
  Logical Operator : Logic  Operator=NOT  AllPortsSameDT=off  OutDataTypeStr=boolean
  Multiport Switch : MultiPortSwitch
  Relational Operator : RelationalOperator  OutDataTypeStr=boolean  RndMeth=Simplest
  AllowTheTankFilling : Outport
  wires:
  Constant/1 -> Multiport Switch/1
  Relational Operator/1 -> Multiport Switch/2
  Constant1/1 -> Multiport Switch/4, Multiport Switch/3
  Multiport Switch/1 -> Logical Operator/1
  Logical Operator/1 -> AllowTheTankFilling/1
  LiquidTank1/1 -> Relational Operator/2
  LiquidTank3/1 -> Relational Operator/1

== system c00014M_harness/M171/Tank3/TankModel ==
  LiquidIn : Inport
  LiquidOut : Inport  Port=2
  Add1 : Sum  Inputs=+-
  Constant1 : Constant  Value=0
  Constant2 : Constant  Value=0
  Constant3 : Constant
  Gain : Gain  Gain=1/R1
  Gain1 : Gain  Gain=1/A1
  Gain2 : Gain  Gain=1/R2
  Integrator : Integrator
  Saturation : Saturate  UpperLimit=hmax  LowerLimit=0
  Switch : Switch  Criteria=u2 ~= 0
  Switch1 : Switch  Criteria=u2 ~= 0
  LiquidLevel : Outport
  wires:
  Saturation/1 -> LiquidLevel/1, Gain2/1
  LiquidOut/1 -> Switch/2
  Add1/1 -> Gain1/1
  Gain2/1 -> Switch/1
  LiquidIn/1 -> Switch1/2
  Switch/1 -> Add1/2
  Switch1/1 -> Gain/1
  Constant2/1 -> Switch/3
  Constant3/1 -> Switch1/1
  Integrator/1 -> Saturation/1
  Gain1/1 -> Integrator/1
  Gain/1 -> Add1/1
  Constant1/1 -> Switch1/3

== system c00014M_harness/M172/Tank1/Control ==
  note: 1: Maintenance
      | 2: Reference
      | 3: Manual
  ControlType : Inport
  Fill : Inport  Port=2
  Empty : Inport  Port=3
  EmergencyButton : Inport  Port=4
  LiquidLevel : Inport  Port=5
  Constant : Constant  Value=0
  ManualControlLiquidInOut : Subsystem
  Switch : Switch  Criteria=u2 > Threshold
  Switch1 : Switch  Criteria=u2 > Threshold
  LiquidIn : Outport
  LiquidOut : Outport  Port=2
  wires:
  LiquidLevel/1 -> ManualControlLiquidInOut/3(LiquidLevel)
  Empty/1 -> ManualControlLiquidInOut/2(Empty)
  Fill/1 -> ManualControlLiquidInOut/1(Fill)
  Switch/1 -> LiquidIn/1
  Switch1/1 -> LiquidOut/1
  Constant/1 -> Switch1/1, Switch/1
  EmergencyButton/1 -> Switch/2, Switch1/2
  ManualControlLiquidInOut/1(LiquidIn) -> Switch/3
  ManualControlLiquidInOut/2(LiquidOut) -> Switch1/3

== system c00014M_harness/M172/Tank1/MasterTankControl ==
  note: Priority tank must always have more liquid than others
  LiquidTank1 : Inport
  LiquidTank3 : Inport  Port=2
  Constant : Constant  Value=PriorityTank
  Constant1 : Constant  Value=false
  Logical Operator : Logic  Operator=NOT  AllPortsSameDT=off  OutDataTypeStr=boolean
  Multiport Switch : MultiPortSwitch
  Relational Operator1 : RelationalOperator  OutDataTypeStr=boolean  RndMeth=Simplest
  AllowTheTankFilling : Outport
  wires:
  LiquidTank3/1 -> Relational Operator1/2
  LiquidTank1/1 -> Relational Operator1/1
  Constant/1 -> Multiport Switch/1
  Relational Operator1/1 -> Multiport Switch/4
  Constant1/1 -> Multiport Switch/2, Multiport Switch/3
  Multiport Switch/1 -> Logical Operator/1
  Logical Operator/1 -> AllowTheTankFilling/1

== system c00014M_harness/M172/Tank1/TankModel ==
  LiquidIn : Inport
  LiquidOut : Inport  Port=2
  Add1 : Sum  Inputs=+-
  Constant1 : Constant  Value=0
  Constant2 : Constant  Value=0
  Constant3 : Constant
  Gain : Gain  Gain=1/R1
  Gain1 : Gain  Gain=1/A1
  Gain2 : Gain  Gain=1/R2
  Integrator : Integrator
  Saturation : Saturate  UpperLimit=hmax  LowerLimit=0
  Switch : Switch  Criteria=u2 ~= 0
  Switch1 : Switch  Criteria=u2 ~= 0
  LiquidLevel : Outport
  wires:
  Saturation/1 -> LiquidLevel/1, Gain2/1
  LiquidOut/1 -> Switch/2
  Add1/1 -> Gain1/1
  Gain2/1 -> Switch/1
  LiquidIn/1 -> Switch1/2
  Switch/1 -> Add1/2
  Switch1/1 -> Gain/1
  Constant2/1 -> Switch/3
  Constant3/1 -> Switch1/1
  Integrator/1 -> Saturation/1
  Gain1/1 -> Integrator/1
  Gain/1 -> Add1/1
  Constant1/1 -> Switch1/3

== system c00014M_harness/M172/Tank3/Control ==
  note: 1: Maintenance
      | 2: Reference
      | 3: Manual
  ControlType : Inport
  StartMaintenance : Inport  Port=2
  EmergencyButton : Inport  Port=3
  LiquidLevel : Inport  Port=4
  Constant : Constant  Value=0
  Maintenance : Subsystem
  Switch : Switch  Criteria=u2 > Threshold
  Switch1 : Switch  Criteria=u2 > Threshold
  LiquidIn : Outport
  LiquidOut : Outport  Port=2
  wires:
  ControlType/1 -> Maintenance/1(Type)
  LiquidLevel/1 -> Maintenance/3(LiquidLevel)
  StartMaintenance/1 -> Maintenance/2(StartMaintenance)
  Switch/1 -> LiquidIn/1
  Switch1/1 -> LiquidOut/1
  Constant/1 -> Switch1/1, Switch/1
  EmergencyButton/1 -> Switch/2, Switch1/2
  Maintenance/1(LiquidIn) -> Switch/3
  Maintenance/2(LiquidOut) -> Switch1/3

== system c00014M_harness/M172/Tank3/MasterTankControl ==
  note: Priority tank must always have more liquid than others
  LiquidTank1 : Inport
  LiquidTank3 : Inport  Port=2
  Constant : Constant  Value=PriorityTank
  Constant1 : Constant  Value=false
  Logical Operator : Logic  Operator=NOT  AllPortsSameDT=off  OutDataTypeStr=boolean
  Multiport Switch : MultiPortSwitch
  Relational Operator : RelationalOperator  OutDataTypeStr=boolean  RndMeth=Simplest
  AllowTheTankFilling : Outport
  wires:
  Constant/1 -> Multiport Switch/1
  Relational Operator/1 -> Multiport Switch/2
  Constant1/1 -> Multiport Switch/4, Multiport Switch/3
  Multiport Switch/1 -> Logical Operator/1
  Logical Operator/1 -> AllowTheTankFilling/1
  LiquidTank1/1 -> Relational Operator/2
  LiquidTank3/1 -> Relational Operator/1

== system c00014M_harness/M172/Tank3/TankModel ==
  LiquidIn : Inport
  LiquidOut : Inport  Port=2
  Add1 : Sum  Inputs=+-
  Constant1 : Constant  Value=0
  Constant2 : Constant  Value=0
  Constant3 : Constant
  Gain : Gain  Gain=1/R1
  Gain1 : Gain  Gain=1/A1
  Gain2 : Gain  Gain=1/R2
  Integrator : Integrator
  Saturation : Saturate  UpperLimit=hmax  LowerLimit=0
  Switch : Switch  Criteria=u2 ~= 0
  Switch1 : Switch  Criteria=u2 ~= 0
  LiquidLevel : Outport
  wires:
  Saturation/1 -> LiquidLevel/1, Gain2/1
  LiquidOut/1 -> Switch/2
  Add1/1 -> Gain1/1
  Gain2/1 -> Switch/1
  LiquidIn/1 -> Switch1/2
  Switch/1 -> Add1/2
  Switch1/1 -> Gain/1
  Constant2/1 -> Switch/3
  Constant3/1 -> Switch1/1
  Integrator/1 -> Saturation/1
  Gain1/1 -> Integrator/1
  Gain/1 -> Add1/1
  Constant1/1 -> Switch1/3

== system c00014M_harness/M173/Tank1/Control ==
  note: 1: Maintenance
      | 2: Reference
      | 3: Manual
  ControlType : Inport
  Fill : Inport  Port=2
  Empty : Inport  Port=3
  EmergencyButton : Inport  Port=4
  LiquidLevel : Inport  Port=5
  Constant : Constant  Value=0
  ManualControlLiquidInOut : Subsystem
  Switch : Switch  Criteria=u2 > Threshold
  Switch1 : Switch  Criteria=u2 > Threshold
  LiquidIn : Outport
  LiquidOut : Outport  Port=2
  wires:
  LiquidLevel/1 -> ManualControlLiquidInOut/3(LiquidLevel)
  Empty/1 -> ManualControlLiquidInOut/2(Empty)
  Fill/1 -> ManualControlLiquidInOut/1(Fill)
  Switch/1 -> LiquidIn/1
  Switch1/1 -> LiquidOut/1
  Constant/1 -> Switch1/1, Switch/1
  EmergencyButton/1 -> Switch/2, Switch1/2
  ManualControlLiquidInOut/1(LiquidIn) -> Switch/3
  ManualControlLiquidInOut/2(LiquidOut) -> Switch1/3
